simulink model "can_simple_block_bu11143"  (R2016b)
settings: Solver=FixedStepDiscrete  StartTime=0.0  StopTime=1000  FixedStep=0.2  RelTol=1e-3  EnableMultiTasking=on
undefined symbols (not defined in the file or in its folder): A, A10, A14, B, B11, B12, B13, B8, C, CS0, CS1, D, D11, D4, F3, F4, G, G3, G4, H3, H4, K17, K4, L3, N16, PA11, PA12, PD0, PE14, PE15, R10, R14, R17, SCK, SIN, SOUT, T14
libraries: rappid_564xl_ec_toolbox x59
(part 2 of 6)

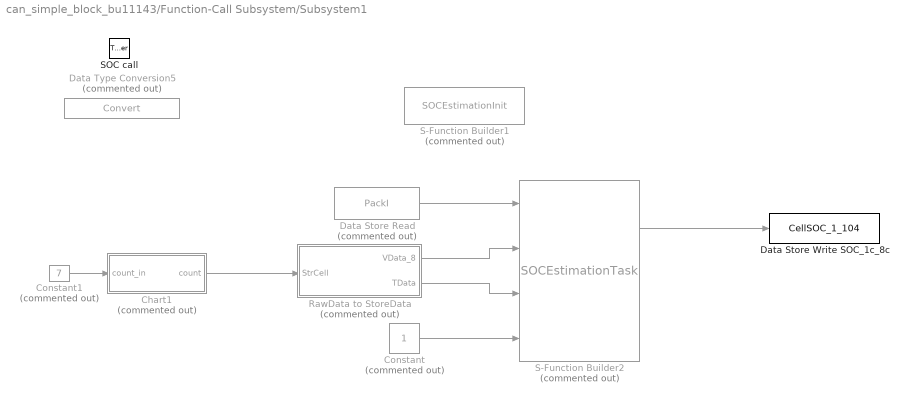
== system can_simple_block_bu11143/Function-Call Subsystem/Subsystem1 ==
  SOC call : TriggerPort  TriggerType=function-call  VariantControl=Variant
  Chart1 : Stateflow chart  Commented=on  TreatAsAtomicUnit=on
  Constant : Constant  Commented=on
  Constant1 : Constant  Commented=on  Value=7  OutDataTypeStr=uint8
  Data Store Read : DataStoreRead  Commented=on  DataStoreName=PackI
  Data Store Write SOC_1c_8c : DataStoreWrite  DataStoreName=CellSOC_1_104
  Data Type Conversion5 : DataTypeConversion  Priority=1  Commented=on
  RawData to StoreData : MATLAB Function  Commented=on  TreatAsAtomicUnit=on
  S-Function Builder1 : S-Function  Commented=on  InitFcn=try, set_param(gcb,'FunctionName','SOCEstimationInit'), end  FunctionName=SOCEstimationInit  SFunctionModules=SOCEstimationInit_wrapper Extended look2_binlx rtGetNaN rtGetInf rt_nonfinite const_params rt_roundd_snf  SFunctionDeploymentMode=off  EnableBusSupport=off  mask(S-Function Builder){}
      mask help: Simulink:masks:SFunctionBuilder_MD
      mask init: same as can_simple_block_bu11143/Function-Call Subsystem/S-Function Builder
      settings: CopyFcn=set_param(gcbh,'LinkStatus','none')  PreSaveFcn=try, set_param(gcb,'FunctionName','SOCEstimationInit'), end  OpenFcn=sfunctionwizard(gcbh)
      mask Display:
      | plot(val(:,1),val(:,2))
      | disp(sys)
  S-Function Builder2 : S-Function  Commented=on  InitFcn=try, set_param(gcb,'FunctionName','SOCEstimationTask'), end  FunctionName=SOCEstimationTask  SFunctionModules=SOCEstimationTask_wrapper Extended look2_binlx rtGetNaN rtGetInf rt_nonfinite const_params rt_roundd_snf  SFunctionDeploymentMode=off  EnableBusSupport=off  mask(S-Function Builder){}
      mask help: Simulink:masks:SFunctionBuilder_MD
      mask init: same as can_simple_block_bu11143/Function-Call Subsystem/S-Function Builder
      settings: CopyFcn=set_param(gcbh,'LinkStatus','none')  PreSaveFcn=try, set_param(gcb,'FunctionName','SOCEstimationTask'), end  OpenFcn=sfunctionwizard(gcbh)
      mask Display: plot(val(:,1),val(:,2)),disp(sys), port_label('input',1,'I'), port_label('input',2,'V8'), port_label('input',3,'T'), port_label('input',4,'Enable8'), port_label('output',1,'SOC'), port_label('output',2,'Vt')
  wires:
  Constant1/1 -> Chart1/1(count_in)
  Chart1/1(count) -> RawData to StoreData/1(StrCell)
  RawData to StoreData/1(VData_8) -> S-Function Builder2/2
  Data Store Read/1 -> S-Function Builder2/1
  RawData to StoreData/2(TData) -> S-Function Builder2/3
  Constant/1 -> S-Function Builder2/4
  S-Function Builder2/1 -> Data Store Write SOC_1c_8c/1

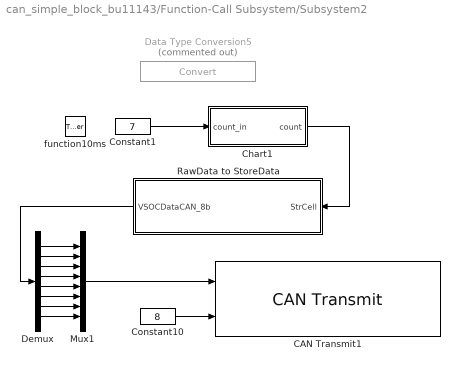
== system can_simple_block_bu11143/Function-Call Subsystem/Subsystem2 ==
  function10ms : TriggerPort  TriggerType=function-call  VariantControl=Variant
  CAN Transmit1 : rappid_564xl_ec_toolbox/MPC564xL/Communication Blocks/CAN Transmit  can_unit=A  can_unit_v2=0  can_buffer=16  can_id=524
  Chart1 : Stateflow chart  TreatAsAtomicUnit=on
  Constant1 : Constant  Value=7  OutDataTypeStr=uint8
  Constant10 : Constant  Value=8  OutDataTypeStr=uint8
  Data Type Conversion5 : DataTypeConversion  Priority=1  Commented=on
  Demux : Demux  Outputs=8
  Mux1 : Mux  Inputs=8
  RawData to StoreData : MATLAB Function  TreatAsAtomicUnit=on
  wires:
  Constant10/1 -> CAN Transmit1/2
  RawData to StoreData/1(VSOCDataCAN_8b) -> Demux/1
  Constant1/1 -> Chart1/1(count_in)
  Chart1/1(count) -> RawData to StoreData/1(StrCell)
  Demux/1 -> Mux1/1
  Demux/2 -> Mux1/2
  Demux/3 -> Mux1/3
  Demux/4 -> Mux1/4
  Demux/5 -> Mux1/5
  Demux/6 -> Mux1/6
  Demux/8 -> Mux1/8
  Demux/7 -> Mux1/7
  Mux1/1 -> CAN Transmit1/1

== system can_simple_block_bu11143/Function-Call Subsystem/Subsystem3 ==
  SPIInitSig : TriggerPort  TriggerType=function-call  VariantControl=Variant
  Constant : Constant  Value=22
  Constant1 : Constant  Value=22
  DSPI Transmit : rappid_564xl_ec_toolbox/MPC564xL/Communication Blocks/DSPI Transmit  Priority=2  dspi_Num=1  dspi_CONT=off  dspi_PUSHR_PE=off  dspi_PUSHR_PP=off  dspi_PCS_0=36 : C[4] : [11] : [H3] : CS0  dspi_PCS_1=105 : G[9] : [79] : [R17] : CS1  dspi_PCS_2=3 : A[3] : [92] : [K17] : CS0  dspi_PCS_slave_0=36 : C[4] : [11] : [H3] : CS0  dspi_PCS_slave_1=5 : A[5] : [14] : [H4] : CS0  dspi_PCS_slave_2=3 : A[3] : [92] : [K17] : CS0  dspi_SIN_0=39 : C[7] : [15] : [K4] : SIN  dspi_SIN_1=8 : A[8] : [12] : [F4]  dspi_SIN_2=2 : A[2] : [84] : [N16] : SIN  dspi_SCK_0=37 : C[5] : [13] : [G3] : SCK  dspi_SCK_1=6 : A[6] : [2] : [G4] : SCK  dspi_SCK_2=0 : A[0] : [73] : [T14] : SCK  dspi_SOUT_0=38 : C[6] : [142] : [D4] : SOUT  dspi_SOUT_1=7 : A[7] : [10] : [F3] : SOUT  dspi_SOUT_2=1 : A[1] : [74] : [R14] : SOUT  dspi_Strobe=None  dspi_eoq=off  dspi_pcsx=Assert
  DSPI Transmit1 : rappid_564xl_ec_toolbox/MPC564xL/Communication Blocks/DSPI Transmit  Priority=2  dspi_Num=1  dspi_CONT=off  dspi_PUSHR_PE=off  dspi_PUSHR_PP=off  dspi_PCS_0=36 : C[4] : [11] : [H3] : CS0  dspi_PCS_1=5 : A[5] : [14] : [H4] : CS0  dspi_PCS_2=3 : A[3] : [92] : [K17] : CS0  dspi_PCS_slave_0=36 : C[4] : [11] : [H3] : CS0  dspi_PCS_slave_1=5 : A[5] : [14] : [H4] : CS0  dspi_PCS_slave_2=3 : A[3] : [92] : [K17] : CS0  dspi_SIN_0=39 : C[7] : [15] : [K4] : SIN  dspi_SIN_1=8 : A[8] : [12] : [F4]  dspi_SIN_2=2 : A[2] : [84] : [N16] : SIN  dspi_SCK_0=37 : C[5] : [13] : [G3] : SCK  dspi_SCK_1=6 : A[6] : [2] : [G4] : SCK  dspi_SCK_2=0 : A[0] : [73] : [T14] : SCK  dspi_SOUT_0=38 : C[6] : [142] : [D4] : SOUT  dspi_SOUT_1=7 : A[7] : [10] : [F3] : SOUT  dspi_SOUT_2=1 : A[1] : [74] : [R14] : SOUT  dspi_Strobe=None  dspi_eoq=off  dspi_pcsx=Assert
  Data Type Conversion : DataTypeConversion  Priority=1
  Data Type Conversion1 : DataTypeConversion  Priority=1
  Pulse Generator7 : DiscretePulseGenerator  Commented=on  Amplitude=0  Period=100
  wires:
  Data Type Conversion/1 -> DSPI Transmit/1
  Constant/1 -> Data Type Conversion/1
  Data Type Conversion1/1 -> DSPI Transmit1/1
  Constant1/1 -> Data Type Conversion1/1

== system can_simple_block_bu11143/Function-Call Subsystem/Subsystem4 ==
  function10ms : TriggerPort  TriggerType=function-call  VariantControl=Variant
  CAN Transmit1 : rappid_564xl_ec_toolbox/MPC564xL/Communication Blocks/CAN Transmit  can_unit=A  can_unit_v2=0  can_buffer=15  can_id=523
  Chart1 : Stateflow chart  TreatAsAtomicUnit=on
  Constant1 : Constant  Value=26  OutDataTypeStr=uint8
  Constant10 : Constant  Value=8  OutDataTypeStr=uint8
  Data Type Conversion5 : DataTypeConversion  Priority=1  Commented=on
  Demux : Demux  Outputs=8
  Mux1 : Mux  Inputs=8
  RawData to StoreData : MATLAB Function  TreatAsAtomicUnit=on
  wires:
  Constant10/1 -> CAN Transmit1/2
  RawData to StoreData/1(VTDataCAN_8b) -> Demux/1
  Constant1/1 -> Chart1/1(count_in)
  Chart1/1(count) -> RawData to StoreData/1(StrCell)
  Demux/1 -> Mux1/1
  Demux/2 -> Mux1/2
  Demux/3 -> Mux1/3
  Demux/4 -> Mux1/4
  Demux/5 -> Mux1/5
  Demux/6 -> Mux1/6
  Demux/8 -> Mux1/8
  Demux/7 -> Mux1/7
  Mux1/1 -> CAN Transmit1/1

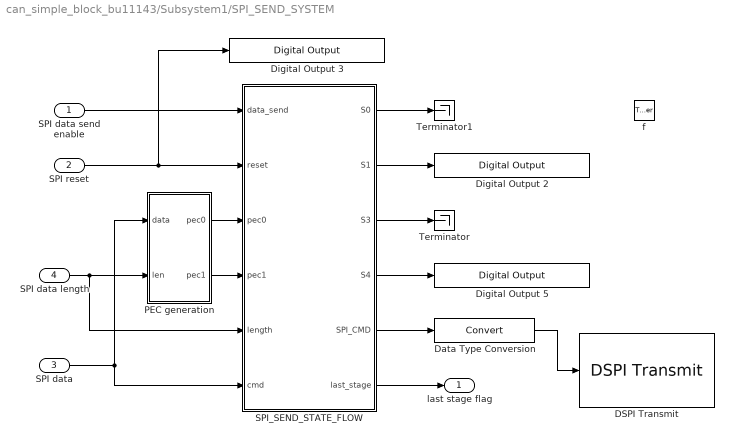
== system can_simple_block_bu11143/Subsystem1/SPI_SEND_SYSTEM ==
  SPI data send enable : Inport
  SPI reset : Inport  Port=2
  SPI data : Inport  Port=3
  SPI data length : Inport  Port=4
  f : TriggerPort  TriggerType=function-call  VariantControl=Variant
  DSPI Transmit : rappid_564xl_ec_toolbox/MPC564xL/Communication Blocks/DSPI Transmit  Priority=2  dspi_Num=1  dspi_CONT=off  dspi_PUSHR_PE=off  dspi_PUSHR_PP=off  dspi_PCS_0=36 : C[4] : [11] : [H3] : CS0  dspi_PCS_1=5 : A[5] : [14] : [H4] : CS0  dspi_PCS_2=3 : A[3] : [92] : [K17] : CS0  dspi_PCS_slave_0=36 : C[4] : [11] : [H3] : CS0  dspi_PCS_slave_1=5 : A[5] : [14] : [H4] : CS0  dspi_PCS_slave_2=3 : A[3] : [92] : [K17] : CS0  dspi_SIN_0=39 : C[7] : [15] : [K4] : SIN  dspi_SIN_1=8 : A[8] : [12] : [F4]  dspi_SIN_2=2 : A[2] : [84] : [N16] : SIN  dspi_SCK_0=37 : C[5] : [13] : [G3] : SCK  dspi_SCK_1=6 : A[6] : [2] : [G4] : SCK  dspi_SCK_2=0 : A[0] : [73] : [T14] : SCK  dspi_SOUT_0=38 : C[6] : [142] : [D4] : SOUT  dspi_SOUT_1=7 : A[7] : [10] : [F3] : SOUT  dspi_SOUT_2=1 : A[1] : [74] : [R14] : SOUT  dspi_Strobe=None  dspi_eoq=off  dspi_pcsx=Assert
  Data Type Conversion : DataTypeConversion  Priority=1
  Digital Output 2 : rappid_564xl_ec_toolbox/MPC564xL/General Purpose Blocks/Digital Output   gpio_outputs="11  : PA11 : [ 120 ] : [ D11 ]"  pinNum=[ 120 ]  pcrNum=11
  Digital Output 3 : rappid_564xl_ec_toolbox/MPC564xL/General Purpose Blocks/Digital Output   gpio_outputs="79  : PE15 : [ 121 ] : [ B11 ]"  pinNum=[ 121 ]  pcrNum=79
  Digital Output 5 : rappid_564xl_ec_toolbox/MPC564xL/General Purpose Blocks/Digital Output   gpio_outputs="48  : PD0  : [ 125 ] : [ B8 ]"  pinNum=[ 125 ]  pcrNum=48
  PEC generation : MATLAB Function  TreatAsAtomicUnit=on
  SPI_SEND_STATE_FLOW : Stateflow chart  TreatAsAtomicUnit=on
  Terminator : Terminator
  Terminator1 : Terminator
  last stage flag : Outport
  wires:
  SPI_SEND_STATE_FLOW/4(" S4") -> Digital Output 5/1
  SPI_SEND_STATE_FLOW/5(SPI_CMD) -> Data Type Conversion/1
  SPI_SEND_STATE_FLOW/1(" S0") -> Terminator1/1
  SPI_SEND_STATE_FLOW/2(" S1") -> Digital Output 2/1
  SPI data send enable/1 -> SPI_SEND_STATE_FLOW/1(data_send)
  SPI reset/1 -> Digital Output 3/1, SPI_SEND_STATE_FLOW/2(reset)
  SPI_SEND_STATE_FLOW/3(" S3") -> Terminator/1
  Data Type Conversion/1 -> DSPI Transmit/1
  SPI_SEND_STATE_FLOW/6(last_stage) -> last stage flag/1
  SPI data/1 -> SPI_SEND_STATE_FLOW/6(cmd), PEC generation/1(data)
  SPI data length/1 -> SPI_SEND_STATE_FLOW/5(length), PEC generation/2(len)
  PEC generation/1(pec0) -> SPI_SEND_STATE_FLOW/3(pec0)
  PEC generation/2(pec1) -> SPI_SEND_STATE_FLOW/4(pec1)

== stateflow chart can_simple_block_bu11143/Subsystem2/Chart ==
  state A
  state A1
  (default) -> A : {count =0;}
  A -> A1
  A1 -> A : { count = count + 1;}
  data: count output uint16; A output boolean

== stateflow chart can_simple_block_bu11143/Subsystem1/Chart ==
  state SENDING
    du:out_sig;
    du:count=count+1;
  state READY
    en:count = 1;
  (default) -> READY : {count=1;}
  READY -> SENDING : {out_sig}
  SENDING -> READY : [count > 3]
  data: start input; last input; count local
  events: out_sig output FUNCTION_CALL_EVENT

== stateflow chart can_simple_block_bu11143/Subsystem3/Chart ==
  state SENDING
    du:out_sig;
  state READY
  (default) -> READY : {count=1;}
  READY -> SENDING : [start == 1]
  SENDING -> READY : [last == 1]
  data: start input; last input; count local
  events: out_sig output FUNCTION_CALL_EVENT

== matlab function can_simple_block_bu11143/Subsystem1/SPI_SEND_SYSTEM/PEC generation ==
  data: data input; len input; pec0 output; pec1 output
function [pec0, pec1]  = PecGen(data,len)

% data_uint8 = uint8(data);
pec15Table = [0 50585 52907 2866 55503 7510 5732 54269 62471 12702 15020 65333 ...
    11464 59729 57955 10234 44439 26638 25404 42661 30040 45249 48115 ... 
    32362 22928 39945 38715	21154	33119	17606	20468	35437	23342	40631	...
    38277	20508	33761	18040	19786	35027	44841	27312	24962	42011	30694	45695	47437	31956	63161	13088	14354	64907	11894	60399	57565	9540	702	50983	52245	2444	55921	8168	5338	53571	62405	13916	15726	63735	11018	61075	58785	8248	1986	49755	51561	3312	57101	6804	4518	54335	24146	39883	37113	21856	34461	17156	18486	36271	43605	28620	25854	41319	29338	46851	48177	31144	43243	28018	26176	41945	28708	46525	48783	31510	23788	39285	37447	22494	33827	16826	19080	36625	1404	49381	52183	3662	56755	6186	4888	54913	61819	13538	16336	64073	10676	60461	59167	8838	41491	26506	27832	43297	31452	48965	46199	29166	22036	37773	39103	23846	36571	19266	16496 ... 
    34281	3972	51741	49455	1206	55115	4818	6624	56441	64387	15898	13608	61617	9036	59093	60903	10366	63805	15524	14230	61967	8690	58475	61273	10944	3386	51363	50065	1544	54773	4204	7006	57031	21674	37171	39425	24472	35941	18940	17102	34647	41133	25908	28166	43935	30818	48635	46793	29520	20950	37967	40829	23268	35097	19584	18354	33323	42449	24648	27514	44771	32030	47239	46005	30252	64577	14808	13034	63347	9358	57623	59941	12220	2118	52703	50925	884	53385	5392	7714	56251	2808	53089	50259	458	53815	6062	7324	55557	65279	15206	12372	62925	9776	58281	59547	11522	42863	25334	27076	44125	32672	47673	45323	29842	21352	38641	40387	22618	35751	20030	17676	32917];
onemask8 = uint16(hex2dec('00FF'));
onemask8_8sft = uint16(hex2dec('FF00'));
onemask88 = uint8(hex2dec('FF'));
onemask16 = uint16(hex2dec('FFFF'));

% data_test = zeros(1,2);
remainder = uint16(16);

for i=1:len
    ii = uint16(i);
%     data_test(1,i) = data(ii);
%     address = 2;
    address = bitand( ...
        bitxor( ...
        uint8(bitsra(remainder,7)),data(ii) ), ...
        onemask88);
    remainder = bitxor(bitshift(remainder,8,'uint16'),pec15Table(address+1));
end
pec15 = uint16(bitand(bitshift(remainder,1,'uint16'),onemask16));
pec0 = uint8(bitand(pec15,onemask8));
pec1 = uint8(bitsra(bitand(pec15,onemask8_8sft),8));

== stateflow chart can_simple_block_bu11143/Subsystem1/SPI_SEND_SYSTEM/SPI_SEND_STATE_FLOW ==
  state S0 [commented out]
    du:last_stage=0;
    en: cmd_i = 1;
  state S1
    en:	cmd_i = 0;
    SPI_CMD=cmd[cmd_i];
    du:
    cmd_i = cmd_i + 1;
    SPI_CMD=cmd[cmd_i];
  state S4
    en:SPI_CMD=pec0;
  state S3
    en:SPI_CMD=pec1;
  S0 -> S1 [commented out] : [data_send == true]
  (default) -> S1 : {count =0;}
  S1 -> S0 [commented out] : [reset == true]
  S4 -> S1 : {last_stage=true;}
  S3 -> S4 [order 1] : [reset == false]
  S3 -> S1 [order 2] : [reset == true]
  S1 -> S1 [order 2] : [reset == true]
  S1 -> S3 [order 1] : after(20,msec)[cmd_i >= length-1 && reset == false]
      | {cmd_i = 1;}
  data: S0 output boolean; data_send input boolean; reset input boolean; S1 output boolean; S3 output boolean; S4 output boolean; SPI_CMD output uint16; count local double; last_stage output boolean; pec0 input uint8; pec1 input uint8; cmd_i local uint8; length input uint8; cmd input uint8

== stateflow chart can_simple_block_bu11143/Chart ==
  state Aoffset
    en:offcnt = 1;
    du:offcnt = offcnt + 1;
  state Aon
    en:testoncnt=1;
    du:testoncnt=testoncnt+1;
    du:out_fcn_call;
  state Aoff
    en:testoffcnt=1;
    du:testoffcnt=testoffcnt+1;
  (default) -> Aoffset : {count =0;}
  Aoffset -> Aon : [offcnt >= off_input]
  Aoff -> Aon : [testoffcnt >= testoff_input]
  Aon -> Aoff : [testoncnt >= teston_input]
  data: count output double; Aoffset output boolean; testcnt local double; off_input input; testoff_input input; teston_input input; offcnt local double; testoffcnt local double; testoncnt local double
  events: out_fcn_call output FUNCTION_CALL_EVENT

== stateflow chart can_simple_block_bu11143/Function-Call Subsystem/Chart ==
  state A
  state A1
  state A2
  (default) -> A : {count =0;}
  A -> A1 : {sig_trigger}
  A2 -> A1
  A1 -> A2 : { count = count + 1;}
  data: count output double [0..10000]; A output boolean [0..1]
  events: sig_trigger output FUNCTION_CALL_EVENT

== matlab function can_simple_block_bu11143/MATLAB Function ==
  data: u input; yh output; yl output
function [yh,yl] = split16to8(u)
onemask8 = uint16(hex2dec('00FF'));
onemask8_8sft = uint16(hex2dec('FF00'));

yl = uint8(bitand(u,onemask8));
yh = uint8(bitsra(bitand(u,onemask8_8sft),8));

== stateflow chart can_simple_block_bu11143/Function-Call Subsystem/Chart2 ==
  state A
    en: count = 0;
    du: count = count + 1;
  state A1
    en: count = 0;
  (default) -> A : {count =0;}
  A -> A1 : [count > count_in]{sig_trigger}
  A1 -> A
  data: count local double [0..10000]; count_in input
  events: sig_trigger output FUNCTION_CALL_EVENT

== matlab function can_simple_block_bu11143/MATLAB Function2 ==
  data: u input; y25_32 output; y17_24 output; y9_16 output; y1_8 output
function [y25_32,y17_24, y9_16,y1_8 ] = split32to8(u)
onemask8 = uint32(hex2dec('000000FF'));
onemask8_8sft = uint32(hex2dec('0000FF00'));
onemask8_16sft = uint32(hex2dec('00FF0000'));
onemask8_24sft = uint32(hex2dec('FF000000'));

y1_8 = uint8(bitand(u,onemask8));
y9_16 = uint8(bitsra(bitand(u,onemask8_8sft),8));
y17_24 = uint8(bitsra(bitand(u,onemask8_16sft),16));
y25_32 = uint8(bitsra(bitand(u,onemask8_24sft),24));

== stateflow chart can_simple_block_bu11143/Subsystem4/Chart ==
  state A
  state A1
  (default) -> A : {count =0;}
  A -> A1
  A1 -> A : { count = count + 1;}
  data: count output double; A output boolean

== matlab function can_simple_block_bu11143/Function-Call Subsystem/PEC generation ==
  data: data input; len input; pec0 output; pec1 output
function [pec0, pec1]  = PecGen(data,len)

% data_uint8 = uint8(data);
pec15Table = [0 50585 52907 2866 55503 7510 5732 54269 62471 12702 15020 65333 ...
    11464 59729 57955 10234 44439 26638 25404 42661 30040 45249 48115 ... 
    32362 22928 39945 38715	21154	33119	17606	20468	35437	23342	40631	...
    38277	20508	33761	18040	19786	35027	44841	27312	24962	42011	30694	45695	47437	31956	63161	13088	14354	64907	11894	60399	57565	9540	702	50983	52245	2444	55921	8168	5338	53571	62405	13916	15726	63735	11018	61075	58785	8248	1986	49755	51561	3312	57101	6804	4518	54335	24146	39883	37113	21856	34461	17156	18486	36271	43605	28620	25854	41319	29338	46851	48177	31144	43243	28018	26176	41945	28708	46525	48783	31510	23788	39285	37447	22494	33827	16826	19080	36625	1404	49381	52183	3662	56755	6186	4888	54913	61819	13538	16336	64073	10676	60461	59167	8838	41491	26506	27832	43297	31452	48965	46199	29166	22036	37773	39103	23846	36571	19266	16496 ... 
    34281	3972	51741	49455	1206	55115	4818	6624	56441	64387	15898	13608	61617	9036	59093	60903	10366	63805	15524	14230	61967	8690	58475	61273	10944	3386	51363	50065	1544	54773	4204	7006	57031	21674	37171	39425	24472	35941	18940	17102	34647	41133	25908	28166	43935	30818	48635	46793	29520	20950	37967	40829	23268	35097	19584	18354	33323	42449	24648	27514	44771	32030	47239	46005	30252	64577	14808	13034	63347	9358	57623	59941	12220	2118	52703	50925	884	53385	5392	7714	56251	2808	53089	50259	458	53815	6062	7324	55557	65279	15206	12372	62925	9776	58281	59547	11522	42863	25334	27076	44125	32672	47673	45323	29842	21352	38641	40387	22618	35751	20030	17676	32917];
onemask8 = uint16(hex2dec('00FF'));
onemask8_8sft = uint16(hex2dec('FF00'));
onemask88 = uint8(hex2dec('FF'));
onemask16 = uint16(hex2dec('FFFF'));

% data_test = zeros(1,2);
remainder = uint16(16);

for i=1:len
    ii = uint16(i);
%     data_test(1,i) = data(ii);
%     address = 2;
    address = bitand( ...
        bitxor( ...
        uint8(bitsra(remainder,7)),data(ii) ), ...
        onemask88);
    remainder = bitxor(  bitshift(remainder,8,'uint16'), pec15Table(address+1)  );
end
pec15 = uint16(bitand(bitshift(remainder,1,'uint16'),onemask16));
pec0 = uint8(bitand(pec15,onemask8));
pec1 = uint8(bitsra(bitand(pec15,onemask8_8sft),8));

== matlab function can_simple_block_bu11143/Function-Call Subsystem/MATLAB Function2 ==
  data: u input; yh output; yl output
function [yh,yl] = split16to8(u)
onemask8 = uint16(hex2dec('00FF'));
onemask8_8sft = uint16(hex2dec('FF00'));

yl = uint8(bitand(u,onemask8));
yh = uint8(bitsra(bitand(u,onemask8_8sft),8));

== matlab function can_simple_block_bu11143/Function-Call Subsystem/MATLAB Function1 ==
  data: pec0_rcv input uint8; pec1_rcv input uint8; y output; pec0_cal input uint8; pec1_cal input uint8
function y = comp(pec0_rcv, pec1_rcv, pec0_cal, pec1_cal)


if pec0_rcv == pec0_cal && pec1_rcv == pec1_cal
  y = 1;
else
  y = 0;  
end

== stateflow chart can_simple_block_bu11143/Function-Call Subsystem/Data collection chart ==
  state Vol_C123
    en:
    CMD32[0] = 0x03;
    CMD32[1] = 0x70;
    CMD32[2] = 0x00;
    CMD32[3] = 0x04;
    STATE = 0;
    ex:
    Sig_Vol_C123;
  state GPIO45_Vref
    en:
    CMD32[0] = 0x04;
    CMD32[1] = 0x60;
    CMD32[2] = 0x00;
    CMD32[3] = 0x0E;
    STATE = 4;
    ex:
    Sig_GP45REF;
  state Vol_C456
    en:
    CMD32[0] = 0x03;
    CMD32[1] = 0x70;
    CMD32[2] = 0x00;
    CMD32[3] = 0x06;
    STATE = 1;
    ex:
    Sig_Vol_C456;
  state GPIO123
    en:
    CMD32[0] = 0x04;
    CMD32[1] = 0x60;
    CMD32[2] = 0x00;
    CMD32[3] = 0x0C;
    STATE = 3;
    ex:
    Sig_GP123;
  state Vol_C789
    en:
    CMD32[0] = 0x03;
    CMD32[1] = 0x70;
    CMD32[2] = 0x00;
    CMD32[3] = 0x08;
    STATE = 2;
    ex:
    Sig_Vol_C789;
  (default) -> Vol_C123 : {count =0;}
  GPIO45_Vref -> Vol_C123 : { count = count + 1;}
  Vol_C123 -> Vol_C456
  GPIO123 -> GPIO45_Vref
  Vol_C456 -> Vol_C789
  Vol_C789 -> GPIO123
  data: count output double [0..10000]; CMD32 output uint8 size=4; STATE output double
  events: Sig_Vol_C123 output FUNCTION_CALL_EVENT; Sig_GP123 output FUNCTION_CALL_EVENT; Sig_GP45REF output FUNCTION_CALL_EVENT; Sig_Vol_C456 output FUNCTION_CALL_EVENT; Sig_Vol_C789 output FUNCTION_CALL_EVENT

== matlab function can_simple_block_bu11143/Function-Call Subsystem/RawData to StoreData ==
  data: STATE input; SPIData input; PecChk input; CellV_1_104 data_store_memory; DataFault output; CellGP_1_78 data_store_memory; V_REF_AUX data_store_memory
function DataFault   = fcnSpiCh0(STATE, SPIData, PecChk)

global CellV_1_104;
global CellGP_1_78;
global V_REF_AUX;
DataFault =  zeros(1,13);

% const int thermistor_ohm_table[231] = {//unit = 0.1Ohm
%                 36850000, 33710000, 30860000, 28270000, 25920000, 23780000, 21820000, 20050000, 18430000, 16950000, // -80 to -71 degC
%                 15600000, 14360000, 13230000, 12200000, 11260000, 10390000,  9599000,  8872000,  8205000,  7592000, // -70 to -61 degC
%                 7029000,  6511000,  6035000,  5597000,  5194000,  4822000,  4479000,  4163000,  3871000,  3602000, // -60 to -51 degC
%                 3353000,  3123000,  2910000,  2713000,  2530000,  2362000,  2205000,  2059000,  1925000,  1800000, // -50 to -41 degC
%                 2398000,  2260000,  2132000,  2011000,  1898000,  1792000,  1693000,  1600000,  1512000,  1430000, // -40 to -31 degC
%                 1352000,  1279000,  1211000,  1146000,  1086000,  1029000,   974900,   924300,   876600,   831600, // -30 to -21 degC
%                   789100,   749100,   711300,   675700,   642000,   610200,   580100,   551700,   524800,   499400, // -20 to -11 degC
%                   475400,   452700,   431100,   410700,   391400,   373100,   355700,   339300,   323700,   308900, // -10 to  -1 degC
%                   294900,   281500,   268900,   256900,   245500,   234600,   224300,   214500,   205200,   196300, //   0 to   9 degC
%                   187900,   179800,   172200,   164900,   157900,   151300,   145000,   139000,   133300,   127900, //  10 to  19 degC
%                   122600,   117700,   112900,   108400,   104100,   100000,    96050,    92270,    88670,    85230, //  20 to  29 degC
%                    81940,    78800,    75790,    72910,    70160,    67520,    65000,    62580,    60260,    58050, //  30 to  39 degC
%                    55920,    53890,    51930,    50060,    48270,    46550,    44890,    43310,    41790,    40330, //  40 to  49 degC
%                    38930,    37580,    36290,    35040,    33850,    32700,    31600,    30540,    29520,    28540, //  50 to  59 degC
%                    27600,    26690,    25820,    24970,    24170,    23390,    22640,    21910,    21220,    20550, //  60 to  69 degC
%                    19900,    19280,    18680,    18100,    17540,    17000,    16480,    15980,    15490,    15030, //  70 to  79 degC
%                    14580,    14140,    13720,    13320,    12930,    12550,    12180,    11830,    11400,    11160, //  80 to  89 degC
%                    10840,    10530,    10230,     9942,     9663,     9393,     9132,     8879,     8634,     8397, //  90 to  99 degC
%                     8168,     7946,     7731,     7523,     7321,     7126,     6936,     6753,     6575,     6403, // 100 to 109 degC
%                     6235,     6073,     5916,     5764,     5616,     5473,     5334,     5199,     5068,     4941, // 110 to 119 degC
%                     4818,     4698,     4582,     4469,     4359,     4253,     4149,     4049,     3951,     3856, // 120 to 129 degC
%                     3764,     3674,     3587,     3503,     3420,     3340,     3263,     3187,     3113,     3042, // 130 to 139 degC
%                     2972,     2904,     2838,     2774,     2712,     2651,     2592,     2534,     2478,     2423, // 140 to 149 degC
%                     2370                                                                                                                                                                                                                                                                                                                                                                  // 150        degC
% };

thermistor_ohm_table = 0.1*[
                36850000, 33710000, 30860000, 28270000, 25920000, 23780000, 21820000, 20050000, 18430000, 16950000, ...// -80 to -71 degC
                15600000, 14360000, 13230000, 12200000, 11260000, 10390000,  9599000,  8872000,  8205000,  7592000, ...// -70 to -61 degC
                7029000,  6511000,  6035000,  5597000,  5194000,  4822000,  4479000,  4163000,  3871000,  3602000, ...// -60 to -51 degC
                3353000,  3123000,  2910000,  2713000,  2530000,  2362000,  2205000,  2059000,  1925000,  1800000, ...// -50 to -41 degC
                2398000,  2260000,  2132000,  2011000,  1898000,  1792000,  1693000,  1600000,  1512000,  1430000, ...// -40 to -31 degC
                1352000,  1279000,  1211000,  1146000,  1086000,  1029000,   974900,   924300,   876600,   831600, ...// -30 to -21 degC
                  789100,   749100,   711300,   675700,   642000,   610200,   580100,   551700,   524800,   499400, ...// -20 to -11 degC
                  475400,   452700,   431100,   410700,   391400,   373100,   355700,   339300,   323700,   308900, ...// -10 to  -1 degC
                  294900,   281500,   268900,   256900,   245500,   234600,   224300,   214500,   205200,   196300, ...//   0 to   9 degC
                  187900,   179800,   172200,   164900,   157900,   151300,   145000,   139000,   133300,   127900, ...//  10 to  19 degC
                  122600,   117700,   112900,   108400,   104100,   100000,    96050,    92270,    88670,    85230,  ...//  20 to  29 degC
                   81940,    78800,    75790,    72910,    70160,    67520,    65000,    62580,    60260,    58050, ...//  30 to  39 degC
                   55920,    53890,    51930,    50060,    48270,    46550,    44890,    43310,    41790,    40330, ...//  40 to  49 degC
                   38930,    37580,    36290,    35040,    33850,    32700,    31600,    30540,    29520,    28540, ...//  50 to  59 degC
                   27600,    26690,    25820,    24970,    24170,    23390,    22640,    21910,    21220,    20550, ...//  60 to  69 degC
                   19900,    19280,    18680,    18100,    17540,    17000,    16480,    15980,    15490,    15030, ...//  70 to  79 degC
                   14580,    14140,    13720,    13320,    12930,    12550,    12180,    11830,    11400,    11160, ...//  80 to  89 degC
                   10840,    10530,    10230,     9942,     9663,     9393,     9132,     8879,     8634,     8397, ...//  90 to  99 degC
                    8168,     7946,     7731,     7523,     7321,     7126,     6936,     6753,     6575,     6403, ...// 100 to 109 degC
                    6235,     6073,     5916,     5764,     5616,     5473,     5334,     5199,     5068,     4941, ...// 110 to 119 degC
                    4818,     4698,     4582,     4469,     4359,     4253,     4149,     4049,     3951,     3856, ...// 120 to 129 degC
                    3764,     3674,     3587,     3503,     3420,     3340,     3263,     3187,     3113,     3042, ...// 130 to 139 degC
                    2972,     2904,     2838,     2774,     2712,     2651,     2592,     2534,     2478,     2423, ...// 140 to 149 degC
                     2370   ]; % // 150        degC



switch STATE
  case 0 % VC123
    for i=1:13
      CellV_1_104(i*8-7) = uint16(SPIData(i*8-7))+uint16(SPIData(i*8-6))*256;
      CellV_1_104(i*8-6) = uint16(SPIData(i*8-5))+uint16(SPIData(i*8-4))*256;
      CellV_1_104(i*8-5) = uint16(SPIData(i*8-3))+uint16(SPIData(i*8-2))*256;
      if (PecChk(i*2-1) == SPIData(i*8-1)) && (PecChk(i*2) == SPIData(i*8))
        DataFault(i) = 1;
      else
        DataFault(i) = 0;
      end
    end
  case 1 % VC456
    for i=1:13
      CellV_1_104(i*8-4) = uint16(SPIData(i*8-7))+uint16(SPIData(i*8-6))*256;
      CellV_1_104(i*8-3) = uint16(SPIData(i*8-5))+uint16(SPIData(i*8-4))*256;
      CellV_1_104(i*8-2) = uint16(SPIData(i*8-3))+uint16(SPIData(i*8-2))*256;
      if (PecChk(i*2-1) == SPIData(i*8-1)) && (PecChk(i*2) == SPIData(i*8))
        DataFault(i) = 1;
      else
        DataFault(i) = 0;
      end
    end    
  case 2 % VC78
    for i=1:13
      CellV_1_104(i*8-1) = uint16(SPIData(i*8-7))+uint16(SPIData(i*8-6))*256;
      CellV_1_104(i*8-0) = uint16(SPIData(i*8-5))+uint16(SPIData(i*8-4))*256;
%       CellV_1_104(i*8-2) = uint16(SPIData(i*8-3))+uint16(SPIData(i*8-2))*256;
      if (PecChk(i*2-1) == SPIData(i*8-1)) && (PecChk(i*2) == SPIData(i*8))
        DataFault(i) = 1;
      else
        DataFault(i) = 0;
      end
    end    
  case 3 % GP123
    V_REF_AUX = uint16(30000);
    for i=1:13
%       v_aux  = int16(uint16(SPIData(i*8-7))+uint16(SPIData(i*8-6))*256);
      v_aux  = (uint16(SPIData(i*8-7))+uint16(SPIData(i*8-6))*256);
      r_tm = (10000*v_aux)/(V_REF_AUX - v_aux);       
%        V_REF_AUX = uint16(30000);
      temperature = (find(thermistor_ohm_table<r_tm,1))-81;
      CellGP_1_78(i*6-5) = v_aux;
      
      v_aux  = (uint16(SPIData(i*8-5))+uint16(SPIData(i*8-4))*256);
      r_tm = (10000*v_aux)/(V_REF_AUX - v_aux);
      temperature = (find(thermistor_ohm_table<r_tm,1))-81;
%        v_aux  = uint16(16000);       
      CellGP_1_78(i*6-4) = v_aux;
      
      v_aux  = (uint16(SPIData(i*8-3))+uint16(SPIData(i*8-2))*256);
      r_tm = (10000*v_aux) / (V_REF_AUX - v_aux);
      temperature = (find(thermistor_ohm_table<r_tm,1))-81;
      CellGP_1_78(i*6-3) = v_aux;      
      if (PecChk(i*2-1) == SPIData(i*8-1)) && (PecChk(i*2) == SPIData(i*8))
        DataFault(i) = 1;
      else
        DataFault(i) = 0;
      end
    end        
  case 4 % GP45
    for i=1:13
      v_aux  = (uint16(SPIData(i*8-7))+uint16(SPIData(i*8-6))*256);
      r_tm = (10000*v_aux)/(V_REF_AUX - v_aux);
      temperature = (find(thermistor_ohm_table<r_tm,1))-81;
      CellGP_1_78(i*6-2) = temperature;
      
      v_aux  = (uint16(SPIData(i*8-5))+uint16(SPIData(i*8-4))*256);
      r_tm = (10000*v_aux)/(V_REF_AUX - v_aux);
      temperature = (find(thermistor_ohm_table<r_tm,1))-81;
      CellGP_1_78(i*6-1) = temperature;      
      
      CellGP_1_78(i*6-0) = uint16(uint16(SPIData(i*8-3))+uint16(SPIData(i*8-2))*256);
      
      V_REF_AUX = (uint16(SPIData(i*8-3))+uint16(SPIData(i*8-2))*256);
      
      if (PecChk(i*2-1) == SPIData(i*8-1)) && (PecChk(i*2) == SPIData(i*8))
        DataFault(i) = 1;
      else
        DataFault(i) = 0;
      end
    end           
  otherwise % ERROR    
end


% CellV_1_104(1) = uint16(1);

% SPIDataStore = uint16(zeros(1,21));
% DataFault =  zeros(1,7);
%
% for i=1:7
%   SPIDataStore(i*3-2) = SPIData(i*8-7)+SPIData(i*8-6)*256;
%   SPIDataStore(i*3-1) = SPIData(i*8-5)+SPIData(i*8-4)*256;
%   SPIDataStore(i*3   ) = SPIData(i*8-3)+SPIData(i*8-2)*256;
%   if (PecChk(i*2-1) == SPIData(i*8-1)) && (PecChk(i*2) == SPIData(i*8))
%     DataFault(i) = 1;
%   else
%     DataFault(i) = 0;
%   end
% end



% onemask8 = uint16(hex2dec('00FF'));
% onemask8_8sft = uint16(hex2dec('FF00'));
% onemask88 = uint8(hex2dec('FF'));
% onemask16 = uint16(hex2dec('FFFF'));
%
% % data_test = zeros(1,2);
% remainder = uint16(16);
%
% for i=1:len
%     ii = uint16(i);
% %     data_test(1,i) = data(ii);
% %     address = 2;
%     address = bitand( ...
%         bitxor( ...
%         uint8(bitsra(remainder,7)),data(ii) ), ...
%         onemask88);
%     remainder = bitxor(bitshift(remainder,8,'uint16'),pec15Table(address+1));
% end
% pec15 = uint16(bitand(bitshift(remainder,1,'uint16'),onemask16));
% pec0 = uint8(bitand(pec15,onemask8));
% pec1 = uint8(bitsra(bitand(pec15,onemask8_8sft),8));

== stateflow chart can_simple_block_bu11143/Function-Call Subsystem/V_DUMP_CAN ==
  state A
    en: count = 0;
    du: count = count + 1;
  state A1
    en: count = 0;
  (default) -> A : {count =0;}
  A -> A1 : [count > count_in]{sig_trigger}
  A1 -> A
  data: count local double [0..10000]; count_in input
  events: sig_trigger output FUNCTION_CALL_EVENT

== matlab function can_simple_block_bu11143/Function-Call Subsystem/Subsystem/RawData to StoreData ==
  data: StrCell input; CellV_1_104 data_store_memory; VTDataCAN_8b output uint8
function VTDataCAN_8b = fcn(StrCell)
global CellV_1_104;
onemask8 = uint16(hex2dec('00FF'));
onemask8_8sft = uint16(hex2dec('FF00'));
onemask8_56sft = uint64(hex2dec('FF'));
% yl = uint8(bitand(u,onemask8));
% yh = uint8(bitsra(bitand(u,onemask8_8sft),8));
% bitshift(remainder,8)  shift left
% bitsra(remainder,8)  shift right



VTDataCAN_8b =  uint8(zeros(1,8));
VTDataCAN_64b =  uint64(zeros(1,1));
VTDataCAN_4data =  uint8(zeros(1,4));

% VTDataCAN_4data(1) = fix(CellV_1_104(StrCell*4-3)/4);
% VTDataCAN_4data(2) = fix(CellV_1_104(StrCell*4-2)/4);
% VTDataCAN_4data(3) = fix(CellV_1_104(StrCell*4-1)/4);
% VTDataCAN_4data(4) = fix(CellV_1_104(StrCell*4-0)/4);

Bid = StrCell;
VTDataCAN_64b = uint64( Bid ) + ...
                            uint64( bitshift(uint64(CellV_1_104(StrCell*4-3)/4),8 ) ) + ...
                            uint64( bitshift(uint64(CellV_1_104(StrCell*4-2)/4),8+14 ))  + ...
                            uint64( bitshift(uint64(CellV_1_104(StrCell*4-1)/4),8+14+14)  )  + ...
                            uint64( bitshift(uint64(CellV_1_104(StrCell*4-0)/4),8+14+14+14) ) ;

VTDataCAN_8b(1) = uint8( bitand(VTDataCAN_64b,onemask8_56sft) );
VTDataCAN_8b(2) = uint8( bitand(bitsra(VTDataCAN_64b,8*1),onemask8_56sft) );
VTDataCAN_8b(3) = uint8( bitand(bitsra(VTDataCAN_64b,8*2),onemask8_56sft) );
VTDataCAN_8b(4) = uint8( bitand(bitsra(VTDataCAN_64b,8*3),onemask8_56sft) );
VTDataCAN_8b(5) = uint8( bitand(bitsra(VTDataCAN_64b,8*4),onemask8_56sft) );
VTDataCAN_8b(6) = uint8( bitand(bitsra(VTDataCAN_64b,8*5),onemask8_56sft) );
VTDataCAN_8b(7) = uint8( bitand(bitsra(VTDataCAN_64b,8*6),onemask8_56sft) );
VTDataCAN_8b(8) = uint8( bitand(bitsra(VTDataCAN_64b,8*7),onemask8_56sft) );

% VTDataCAN_8b(1) = Bid;
% VTDataCAN_8b(2) = VTDataCAN_4data(1)/(2^8);
% VTDataCAN_8b(3) = 4*fix(mod(CellV_1_104(StrCell*4-3),2^8)/4);
% VTDataCAN_8b(3) = VTDataCAN_8b(3) + CellV_1_104(StrCell*4-2)/(2^14);
% VTDataCAN_8b(4) = mod(CellV_1_104(StrCell*4-2),2^14) / (2^8);
% VTDataCAN_8b(5) =  * fix(mod(CellV_1_104(StrCell*4-2),2^6));

4*fix(CellV_1_104(StrCell*4-3)/4);


% VTDataCAN_8b(1) =         CellV_1_104(StrCell*4-3)/256;
% VTDataCAN_8b(2) = mod(CellV_1_104(StrCell*4-3),256);
% VTDataCAN_8b(3) =         CellV_1_104(StrCell*4-2)/256;
% VTDataCAN_8b(4) = mod(CellV_1_104(StrCell*4-2),256);
% VTDataCAN_8b(5) =         CellV_1_104(StrCell*4-1)/256;
% VTDataCAN_8b(6) = mod(CellV_1_104(StrCell*4-1),256);
% VTDataCAN_8b(7) =         CellV_1_104(StrCell*4   )/256;
% VTDataCAN_8b(8) = mod(CellV_1_104(StrCell*4   ),256);

% VTDataCAN_8b(1) =         CellV_1_104(1)/256;
% VTDataCAN_8b(2) = mod(CellV_1_104(1),256);
% VTDataCAN_8b(3) =         CellV_1_104(2)/256;
% VTDataCAN_8b(4) = mod(CellV_1_104(2),256);
% VTDataCAN_8b(5) =         CellV_1_104(9)/256;
% VTDataCAN_8b(6) = mod(CellV_1_104(9),256);
% VTDataCAN_8b(7) =         CellV_1_104(10)/256;
% VTDataCAN_8b(8) = mod(CellV_1_104(10),256);

% VTDataCAN_8b(1) =         uint16(30000)/256;
% VTDataCAN_8b(2) = mod(uint16(30000),256);
% VTDataCAN_8b(3) =         uint16(35000)/256;
% VTDataCAN_8b(4) = mod(uint16(35000),256);
% VTDataCAN_8b(5) =         uint16(33000)/256;
% VTDataCAN_8b(6) = mod(uint16(33000),256);
% VTDataCAN_8b(7) =         uint16(20000)/256;
% VTDataCAN_8b(8) = mod(uint16(20000),256);


end








% CellV_1_104(1) = uint16(1);

% SPIDataStore = uint16(zeros(1,21));
% DataFault =  zeros(1,7);
%
% for i=1:7
%   SPIDataStore(i*3-2) = SPIData(i*8-7)+SPIData(i*8-6)*256;
%   SPIDataStore(i*3-1) = SPIData(i*8-5)+SPIData(i*8-4)*256;
%   SPIDataStore(i*3   ) = SPIData(i*8-3)+SPIData(i*8-2)*256;
%   if (PecChk(i*2-1) == SPIData(i*8-1)) && (PecChk(i*2) == SPIData(i*8))
%     DataFault(i) = 1;
%   else
%     DataFault(i) = 0;
%   end
% end



% onemask8 = uint16(hex2dec('00FF'));
% onemask8_8sft = uint16(hex2dec('FF00'));
% onemask88 = uint8(hex2dec('FF'));
% onemask16 = uint16(hex2dec('FFFF'));
%
% % data_test = zeros(1,2);
% remainder = uint16(16);
%
% for i=1:len
%     ii = uint16(i);
% %     data_test(1,i) = data(ii);
% %     address = 2;
%     address = bitand( ...
%         bitxor( ...
%         uint8(bitsra(remainder,7)),data(ii) ), ...
%         onemask88);
%     remainder = bitxor(bitshift(remainder,8,'uint16'),pec15Table(address+1));
% end
% pec15 = uint16(bitand(bitshift(remainder,1,'uint16'),onemask16));
% pec0 = uint8(bitand(pec15,onemask8));
% pec1 = uint8(bitsra(bitand(pec15,onemask8_8sft),8));

== stateflow chart can_simple_block_bu11143/Function-Call Subsystem/Subsystem/Chart1 ==
  state A
    en: count  = count + 1;
    du: count = count + 1;
  state A1
    en: count = 1;
  (default) -> A : {count =0;}
  A1 -> A
  A -> A1 : [count >= count_in]
  data: count_in input; count output double [0..10000]

== stateflow chart can_simple_block_bu11143/Function-Call Subsystem/Subsystem1/Chart1 ==
  state A
    en: count  = count + 1;
    du: count = count + 1;
  state A1
    en: count = 1;
  (default) -> A : {count =0;}
  A1 -> A
  A -> A1 : [count >= count_in]
  data: count_in input; count output double [0..10000]

== matlab function can_simple_block_bu11143/Function-Call Subsystem/Subsystem1/RawData to StoreData ==
  data: StrCell input; CellV_1_104 data_store_memory; VData_8 output uint8; TData output
function [VData_8,TData] = fcn(StrCell)

global CellV_1_104;
global CellGP_1_78;

VData_8 =  uint16(zeros(1,8));

VData_8(1) = CellV_1_104(StrCell*8-7);
VData_8(2) = CellV_1_104(StrCell*8-6);
VData_8(3) = CellV_1_104(StrCell*8-5);
VData_8(4) = CellV_1_104(StrCell*8-4);
VData_8(5) = CellV_1_104(StrCell*8-3);
VData_8(6) = CellV_1_104(StrCell*8-2);
VData_8(7) = CellV_1_104(StrCell*8-1);
VData_8(8) = CellV_1_104(StrCell*8   );
TData = 0.2*( CellGP_1_78(StrCell*5-4)+CellGP_1_78(StrCell*5-3) ...
  +CellGP_1_78(StrCell*5-2)+CellGP_1_78(StrCell*5-1)+CellGP_1_78(StrCell*5) );

% VTDataCAN_8b(1) =         CellV_1_104(1)/256;
% VTDataCAN_8b(2) = mod(CellV_1_104(1),256);
% VTDataCAN_8b(3) =         CellV_1_104(2)/256;
% VTDataCAN_8b(4) = mod(CellV_1_104(2),256);
% VTDataCAN_8b(5) =         CellV_1_104(9)/256;
% VTDataCAN_8b(6) = mod(CellV_1_104(9),256);
% VTDataCAN_8b(7) =         CellV_1_104(10)/256;
% VTDataCAN_8b(8) = mod(CellV_1_104(10),256);

% VTDataCAN_8b(1) =         uint16(30000)/256;
% VTDataCAN_8b(2) = mod(uint16(30000),256);
% VTDataCAN_8b(3) =         uint16(35000)/256;
% VTDataCAN_8b(4) = mod(uint16(35000),256);
% VTDataCAN_8b(5) =         uint16(33000)/256;
% VTDataCAN_8b(6) = mod(uint16(33000),256);
% VTDataCAN_8b(7) =         uint16(20000)/256;
% VTDataCAN_8b(8) = mod(uint16(20000),256);


end








% CellV_1_104(1) = uint16(1);

% SPIDataStore = uint16(zeros(1,21));
% DataFault =  zeros(1,7);
%
% for i=1:7
%   SPIDataStore(i*3-2) = SPIData(i*8-7)+SPIData(i*8-6)*256;
%   SPIDataStore(i*3-1) = SPIData(i*8-5)+SPIData(i*8-4)*256;
%   SPIDataStore(i*3   ) = SPIData(i*8-3)+SPIData(i*8-2)*256;
%   if (PecChk(i*2-1) == SPIData(i*8-1)) && (PecChk(i*2) == SPIData(i*8))
%     DataFault(i) = 1;
%   else
%     DataFault(i) = 0;
%   end
% end



% onemask8 = uint16(hex2dec('00FF'));
% onemask8_8sft = uint16(hex2dec('FF00'));
% onemask88 = uint8(hex2dec('FF'));
% onemask16 = uint16(hex2dec('FFFF'));
%
% % data_test = zeros(1,2);
% remainder = uint16(16);
%
% for i=1:len
%     ii = uint16(i);
% %     data_test(1,i) = data(ii);
% %     address = 2;
%     address = bitand( ...
%         bitxor( ...
%         uint8(bitsra(remainder,7)),data(ii) ), ...
%         onemask88);
%     remainder = bitxor(bitshift(remainder,8,'uint16'),pec15Table(address+1));
% end
% pec15 = uint16(bitand(bitshift(remainder,1,'uint16'),onemask16));
% pec0 = uint8(bitand(pec15,onemask8));
% pec1 = uint8(bitsra(bitand(pec15,onemask8_8sft),8));

== stateflow chart can_simple_block_bu11143/Function-Call Subsystem/Chart3 ==
  state InitDMA
    en: sig_DMAInit_trigger;
    du: count = count + 1;
  state DMA_Running
    en: count = 0;
  (default) -> InitDMA : {count =0;}
  InitDMA -> DMA_Running
  DMA_Running -> InitDMA : [DMA_RST == 1]
  data: count local double [0..10000]; count_in input; DMA_RST input
  events: sig_DMAInit_trigger output FUNCTION_CALL_EVENT

== stateflow chart can_simple_block_bu11143/Function-Call Subsystem/Chart4 ==
  state InitDMA
    en: sig_KFInit_trigger;
    du: count = count + 1;
  state DMA_Rest
    en: count = 0;
    du: count = count + 1;
  state DMA_Running
    en: count = 0;
  (default) -> InitDMA : {count =0;}
  InitDMA -> DMA_Rest
  DMA_Running -> InitDMA : [KF_RST == 1]
  DMA_Rest -> InitDMA [order 1] : [KF_RST == 1]
  DMA_Rest -> DMA_Running [order 2] : [count > count_in]{sig_KF_trigger}
  data: count local double [0..10000]; count_in input; KF_RST input
  events: sig_KFInit_trigger output FUNCTION_CALL_EVENT; sig_KF_trigger output FUNCTION_CALL_EVENT

== stateflow chart can_simple_block_bu11143/Function-Call Subsystem/SOCKF_Run/Chart1 ==
  state A
    en: count  = count + 1;
    du: count = count + 1;
  state A1
    en: count = 1;
  (default) -> A : {count =0;}
  A1 -> A
  A -> A1 : [count >= count_in]
  data: count_in input; count output double [0..10000]

== matlab function can_simple_block_bu11143/Function-Call Subsystem/SOCKF_Run/RawData to StoreData ==
  data: StrCell input; CellV_1_104 data_store_memory; VData_8 output uint16; TData output; CellGP_1_78 data_store_memory
function [VData_8,TData] = fcn(StrCell)

global CellV_1_104;
global CellGP_1_78;

VData_8 =  uint16(zeros(1,8));

VData_8(1) = CellV_1_104(StrCell*8-7);
VData_8(2) = CellV_1_104(StrCell*8-6);
VData_8(3) = CellV_1_104(StrCell*8-5);
VData_8(4) = CellV_1_104(StrCell*8-4);
VData_8(5) = CellV_1_104(StrCell*8-3);
VData_8(6) = CellV_1_104(StrCell*8-2);
VData_8(7) = CellV_1_104(StrCell*8-1);
VData_8(8) = CellV_1_104(StrCell*8   );
TData = 0.2*( CellGP_1_78(StrCell*5-4)+CellGP_1_78(StrCell*5-3) ...
  +CellGP_1_78(StrCell*5-2)+CellGP_1_78(StrCell*5-1)+CellGP_1_78(StrCell*5) );

% VTDataCAN_8b(1) =         CellV_1_104(1)/256;
% VTDataCAN_8b(2) = mod(CellV_1_104(1),256);
% VTDataCAN_8b(3) =         CellV_1_104(2)/256;
% VTDataCAN_8b(4) = mod(CellV_1_104(2),256);
% VTDataCAN_8b(5) =         CellV_1_104(9)/256;
% VTDataCAN_8b(6) = mod(CellV_1_104(9),256);
% VTDataCAN_8b(7) =         CellV_1_104(10)/256;
% VTDataCAN_8b(8) = mod(CellV_1_104(10),256);

% VTDataCAN_8b(1) =         uint16(30000)/256;
% VTDataCAN_8b(2) = mod(uint16(30000),256);
% VTDataCAN_8b(3) =         uint16(35000)/256;
% VTDataCAN_8b(4) = mod(uint16(35000),256);
% VTDataCAN_8b(5) =         uint16(33000)/256;
% VTDataCAN_8b(6) = mod(uint16(33000),256);
% VTDataCAN_8b(7) =         uint16(20000)/256;
% VTDataCAN_8b(8) = mod(uint16(20000),256);


end








% CellV_1_104(1) = uint16(1);

% SPIDataStore = uint16(zeros(1,21));
% DataFault =  zeros(1,7);
%
% for i=1:7
%   SPIDataStore(i*3-2) = SPIData(i*8-7)+SPIData(i*8-6)*256;
%   SPIDataStore(i*3-1) = SPIData(i*8-5)+SPIData(i*8-4)*256;
%   SPIDataStore(i*3   ) = SPIData(i*8-3)+SPIData(i*8-2)*256;
%   if (PecChk(i*2-1) == SPIData(i*8-1)) && (PecChk(i*2) == SPIData(i*8))
%     DataFault(i) = 1;
%   else
%     DataFault(i) = 0;
%   end
% end



% onemask8 = uint16(hex2dec('00FF'));
% onemask8_8sft = uint16(hex2dec('FF00'));
% onemask88 = uint8(hex2dec('FF'));
% onemask16 = uint16(hex2dec('FFFF'));
%
% % data_test = zeros(1,2);
% remainder = uint16(16);
%
% for i=1:len
%     ii = uint16(i);
% %     data_test(1,i) = data(ii);
% %     address = 2;
%     address = bitand( ...
%         bitxor( ...
%         uint8(bitsra(remainder,7)),data(ii) ), ...
%         onemask88);
%     remainder = bitxor(bitshift(remainder,8,'uint16'),pec15Table(address+1));
% end
% pec15 = uint16(bitand(bitshift(remainder,1,'uint16'),onemask16));
% pec0 = uint8(bitand(pec15,onemask8));
% pec1 = uint8(bitsra(bitand(pec15,onemask8_8sft),8));

== matlab function can_simple_block_bu11143/Function-Call Subsystem/SOCKF_Run/RawData to StoreData1 ==
  data: StrCell input; CellSOC_1_104 data_store_memory; SOCEsti input
function fcn(StrCell,SOCEsti)

global CellSOC_1_104;

      CellSOC_1_104(StrCell*8-7) = SOCEsti(1);
      CellSOC_1_104(StrCell*8-6) = SOCEsti(2);
      CellSOC_1_104(StrCell*8-5) = SOCEsti(3);
      CellSOC_1_104(StrCell*8-4) = SOCEsti(4);
      CellSOC_1_104(StrCell*8-3) = SOCEsti(5);
      CellSOC_1_104(StrCell*8-2) = SOCEsti(6);
      CellSOC_1_104(StrCell*8-1) = SOCEsti(7);
      CellSOC_1_104(StrCell*8-0) = SOCEsti(8);

end


% CellV_1_104(1) = uint16(1);

% SPIDataStore = uint16(zeros(1,21));
% DataFault =  zeros(1,7);
%
% for i=1:7
%   SPIDataStore(i*3-2) = SPIData(i*8-7)+SPIData(i*8-6)*256;
%   SPIDataStore(i*3-1) = SPIData(i*8-5)+SPIData(i*8-4)*256;
%   SPIDataStore(i*3   ) = SPIData(i*8-3)+SPIData(i*8-2)*256;
%   if (PecChk(i*2-1) == SPIData(i*8-1)) && (PecChk(i*2) == SPIData(i*8))
%     DataFault(i) = 1;
%   else
%     DataFault(i) = 0;
%   end
% end



% onemask8 = uint16(hex2dec('00FF'));
% onemask8_8sft = uint16(hex2dec('FF00'));
% onemask88 = uint8(hex2dec('FF'));
% onemask16 = uint16(hex2dec('FFFF'));
%
% % data_test = zeros(1,2);
% remainder = uint16(16);
%
% for i=1:len
%     ii = uint16(i);
% %     data_test(1,i) = data(ii);
% %     address = 2;
%     address = bitand( ...
%         bitxor( ...
%         uint8(bitsra(remainder,7)),data(ii) ), ...
%         onemask88);
%     remainder = bitxor(bitshift(remainder,8,'uint16'),pec15Table(address+1));
% end
% pec15 = uint16(bitand(bitshift(remainder,1,'uint16'),onemask16));
% pec0 = uint8(bitand(pec15,onemask8));
% pec1 = uint8(bitsra(bitand(pec15,onemask8_8sft),8));

== stateflow chart can_simple_block_bu11143/Function-Call Subsystem/Chart5 ==
  state A
    en: count = 0;
    du: count = count + 1;
  state A1
    en: count = 0;
  (default) -> A : {count =0;}
  A -> A1 : [count > count_in]{sig_trigger}
  A1 -> A
  data: count local double [0..10000]; count_in input
  events: sig_trigger output FUNCTION_CALL_EVENT

== stateflow chart can_simple_block_bu11143/Function-Call Subsystem/Subsystem2/Chart1 ==
  state A
    en: count  = count + 1;
    du: count = count + 1;
  state A1
    en: count = 1;
  (default) -> A : {count =0;}
  A1 -> A
  A -> A1 : [count >= count_in]
  data: count_in input; count output double [0..10000]
